simulink model "AreaCoverageTestHarness"  (R2016b)
settings: Solver=FixedStepDiscrete  StartTime=0.0  StopTime=1000  FixedStep=0.0001  RelTol=1e-3  EnableMultiTasking=on
StopFcn:
  | if strcmp(get_param('AreaCoverageTestHarness/Robot/DetailedMap', 'Commented'), 'off')
  | evalin('base', 'MapCoveragePercent(roomSim)');
  | disp('STOP');
  | end
values from neighbouring files (symbols this model uses):
  BLOCK_SIZE = double(CAL_BLOCK_SIZE)    [AreaCoverageCalib.m]    (also in room_V1.m = 20; room_V2.m = 20; room_V3.m = 20)
  CAL_B_NmPerW = 1.5    [MotorConfigurationSheet.m]
  CAL_CurrentScaling_A = 0.04    [MotorConfigurationSheet.m]
  CAL_flux_e = 0.3    [MotorConfigurationSheet.m]
  CAL_flux_t = 3.0    (= 3)    [MotorConfigurationSheet.m]
  CAL_Inertia_J = 0.03    [MotorConfigurationSheet.m]
  CAL_Re_ohm = 0.5    [MotorConfigurationSheet.m]
  CAL_SimInduct_H = 0.001    [MotorConfigurationSheet.m]
  EAST = 0    [AreaCoverageCalib.m]
  ERRVAL = 5    [AreaCoverageCalib.m]
  gearRatio = 12    [AreaCoverageCalib.m]
  halfWheel_mm = 60    [AreaCoverageCalib.m]
  initXSim = 38    [AreaCoverageCalib.m]
  initYSim = 50    [AreaCoverageCalib.m]
  NORTH = 270    [AreaCoverageCalib.m]
  NVM_AngleStoreFlg = true    [AreaCoverageCalib.m]
  NVM_EAST = uint16(CAL_EAST)    [AreaCoverageCalib.m]
  NVM_NORTH = uint16(CAL_NORTH)    [AreaCoverageCalib.m]
  NVM_SOUTH = uint16(CAL_SOUTH)    [AreaCoverageCalib.m]
  NVM_WEST = uint16(CAL_WEST)    [AreaCoverageCalib.m]
  ROB_LENG_m = 0.25    [AreaCoverageCalib.m]
  ROBO_LENG = 30    [realMapPlotter.m]    (also in roomDrawing.m)
  ROOM_SIDE_SIZE = double(CAL_ROOM_SIDE_SIZE)    [AreaCoverageCalib.m]    (also in room_V1.m = 20; room_V2.m = 20; room_V3.m = 20)
  SAMPLE_TIME = 0.001    [AreaCoverageCalib.m]
  SOUTH = 90    [AreaCoverageCalib.m]
  thetaMapBp = [0 : 0.1 : 360]    [AreaCoverageCalib.m]
  thetaMapTb = [thetaMapTb1, thetaMapTb2, thetaMapTb3, thetaMapTb4, thetaMapTb5]    [AreaCoverageCalib.m]
  WEST = 180    [AreaCoverageCalib.m]
undefined symbols (not defined in the file or in its folder): CAL_WheelDiameter_cm, DiscIntNeverNeededParam, ENU_BACKWARD, ENU_FORWARD
libraries: simulink x3, RobotControlLib x1
(part 3 of 3)

== matlab function AreaCoverageTestHarness/Robot/DetailedMap/createMap/RoomV2/Room_V2 ==
  data: roomOut output size=[ROOM_SIDE_SIZE*BLOCK_SIZE/4 ROOM_SIDE_SIZE*BLOCK_SIZE/4] [0..255]; ROOM_SIDE_SIZE parameter; BLOCK_SIZE parameter
function roomOut = fcn(ROOM_SIDE_SIZE, BLOCK_SIZE)

persistent flag;
persistent room;
   side_size = ROOM_SIDE_SIZE * (BLOCK_SIZE/4);

if isempty(flag)
    flag = false;
    room = uint8(ones(side_size , side_size)*255);
end

if flag == false
   flag = true;
%     room = uint8(ones(ROOM_SIDE_SIZE , ROOM_SIDE_SIZE)*255);

    %% Draw room Boarders
    for rowNum = 1:(side_size)
        for colNum = 1: side_size
            if (rowNum <= BLOCK_SIZE/4) || (rowNum >= (side_size - BLOCK_SIZE/4))...
                    || (colNum <= BLOCK_SIZE/4) || (colNum >= side_size - BLOCK_SIZE/4)
    %                 || (rowNum == 2) || (rowNum == roomSize - 1)...
    %                 || (colNum == 2) || (colNum == roomSize-1)
                room(rowNum, colNum) = 0;
            end
        end
    end

    %% Draw room Obsticals
    scale = 5;
    %% insert Table
    room((14*scale - scale/2) + 0.5:(19*scale + scale/2) + 0.5, (4*scale - scale/4) + 0.5:(4*scale + scale/4 )+ 0.5) = 0;
    room((14*scale - scale/2) + 0.5:(19*scale + scale/2) + 0.5, (6*scale - scale/4) + 0.5:(6*scale + scale/4 )+ 0.5) = 0;
    room((14*scale - scale/2) + 0.5:(19*scale + scale/2) + 0.5, (8*scale - scale/4) + 0.5:(8*scale + scale/4 )+ 0.5) = 0;
    room((14*scale - scale/2) + 0.5:(19*scale + scale/2) + 0.5, (10*scale - scale/4) + 0.5:(10*scale + scale/4 )+ 0.5) = 0;
    room((14*scale - scale/2) + 0.5:(19*scale + scale/2) + 0.5, (12*scale - scale/4) + 0.5:(12*scale + scale/4 )+ 0.5) = 0;
    room((18.5*scale - scale/2) + 0.5:(19*scale + scale/2) + 0.5, (14*scale - scale/2) + 0.5:(14*scale + scale/2 )+ 0.5) = 0;

    %% insert box

    room((10*scale - scale/2) + 0.5:(19*scale + scale/2) + 0.5, (1*scale - (scale)/2) + 0.5:(3*scale + (scale)/2 )+ 0.5) = 0;

    %% insert soffa
    room((1*scale - scale/2) + 0.5:(4*scale + scale/2) + 0.5, (8*scale - (scale)/2) + 0.5:(19*scale + (scale)/2 )+ 0.5) = 0;

    %% insert LeglessTable
    room((7*scale - scale/2) + 0.5:(11*scale + scale/2) + 0.5, (1*scale - scale/2) + 0.5:(4*scale + scale/2 )+ 0.5) = 0;
    
    room((4*scale - scale/2) + 0.5:(19*scale + scale/2) + 0.5, (16*scale - scale/2) + 0.5:(19*scale + scale/2 )+ 0.5) = 0;

    
    roomOut = room;
else
    roomOut = room;
end

== stateflow chart AreaCoverageTestHarness/Robot/OrientationCalculator/VelocityCalculator/LeftPhysicalMotorModel/PulseGenerator/Chart2 ==
  state holdValue
  state updateValue
    en:
    pulseFlg = true;
    ex:
  (default) -> holdValue : /tempTheta = currentTheta;
  holdValue -> updateValue [order 1] : [((tempTheta - currentTheta) >= ((2*pi)/CAL_SingleTurnTicks))...
      | && currentTheta > 0]
      | /debugCounter--;
      | tempTheta = debugCounter*((2*pi)/CAL_SingleTurnTicks);
  holdValue -> updateValue [order 2] : [((tempTheta - currentTheta) < -((2*pi)/CAL_SingleTurnTicks))...
      | && currentTheta > 0]
      | /debugCounter++;
      | tempTheta = debugCounter*((2*pi)/CAL_SingleTurnTicks);
  updateValue -> holdValue : [after(11, tick)]/pulseFlg = false;
  data: CAL_SingleTurnTicks constant single =CAL_SingleTurnTicks; currentTheta input; pulseFlg output boolean; tempTheta local single; pi constant double =pi; debugCounter local uint32
